simulink model "SR25"  (R2024a)
settings: Solver=FixedStepDiscrete  StartTime=0.0  StopTime=5  FixedStep=0.01  RelTol=1e-3  EnableMultiTasking=on
PreLoadFcn:
  | try, model_open; catch, disp('Error occurred while executing model pre-load callback: model_open.m'); disp('Please assure that the MATLAB working directory is set to the model directory before opening.'); end
InitFcn:
  | try, model_open; catch, end
undefined symbols (not defined in the file or in its folder): dt, GCM, raptor_get_safe_string, raptor_xcp_function
libraries: Raptor_lib x40, Utilities x13, TireTemperature x12, simulink x5, IO x5, APPS_BSPC x4, RotorTemperature x4, FlowRate x3, Cooling x2, BMS x2, Brakes x2, StateMachine x2
(part 1 of 3)
CloseFcn:
  | try, model_close; catch, end
settings Model: DataDictionary=SR25.sldd  Raptor_Target=GCM-1793-196-1503  Raptor_Calloc=NonVolatile (EEPROM)  RaptorUIDSize=4  RaptorBuildNum=100  Raptor_ecuaddr=11  Raptor_IsLiteMode=0  RaptorFaultManager=Standard  RaptorFaultManagerAddXYCounts=1  Creator=Ben  LastModifiedBy=msufs
settings SolverCC: AlgebraicLoopSolver=TrustRegion
settings DataIOCC: LimitDataPoints=on  SaveFormat=Array  SignalLoggingSaveFormat=ModelDataLogs  ReturnWorkspaceOutputs=off
settings OptimizationCC: DefaultParameterBehavior=Inlined  DefaultUnderspecifiedDataType=single  ReuseModelBlockBuffer=off  ExpressionDepthLimit=2147483647  InitFltsAndDblsToZero=on  LifeSpan=1  EfficientTunableParamExpr=on
settings DebuggingCC: SolverPrmCheckMsg=warning  InheritedTsInSrcMsg=none  FcnCallInpInsideContextMsg=warning  UnconnectedInputMsg=warning  UnconnectedOutputMsg=warning  UnconnectedLineMsg=warning  StateNameClashWarn=warning  SFUnexpectedBacktrackingDiag=warning  SFNoUnconditionalDefaultTransitionDiag=warning  SFExecutionAtInitializationDiag=none  ArithmeticOperatorsInVariantConditions=warning
settings HardwareCC: ProdBitPerPointer=32  ProdBitPerSizeT=32  ProdBitPerPtrDiffT=32  ProdLargestAtomicFloat=None  ProdWordSize=32  ProdHWDeviceType=Infineon->TriCore  TargetIntDivRoundTo=Zero  TargetEndianess=LittleEndian  TargetHWDeviceType=Infineon->TriCore  ProdEqTarget=off
settings ModelReferenceCC: EnableRefExpFcnMdlSchedulingChecks=on  PropagateSignalLabelsOutOfModel=off
settings SFSimCC: SimUseLocalCustomCode=off  MATLABDynamicMemAlloc=off  CustomCodeUndefinedFunction=UseInterfaceOnly
settings RTWCC: Description=Raptor (tm)  SystemTargetFile=raptor.tlc  MakeCommand=raptor_make_rtw  TemplateMakefile=raptor_GCM_1793_196_GCC.tmf  RTWUseLocalCustomCode=off  GPUComputeCapability=3.5
settings CodeAppCC: IgnoreCustomStorageClasses=off  MaxIdLength=100  CustomSymbolStrType=$N$R$M  StateflowObjectComments=on  InternalIdentifier=Classic
settings STFCustomTargetCC: TargetLangStandard=C89/C90 (ANSI)  CodeReplacementLibrary=GCM196-specific  GenerateSampleERTMain=on  CombineOutputUpdateFcns=on  ERTCustomFileBanners=on  SupportContinuousTime=off  SupportNonInlinedSFcns=off  RemoveResetFunc=on  MATLABClassNameForMDSCustomization=Simulink.SoftwareTarget.ERTCustomization  GRTInterface=off  UseToolchainInfoCompliant=off  SystemTargetFile=raptor.tlc
settings ERTTargetCC: CodeReplacementLibrary=GCM196-specific  MultiwordLength=2048  GenerateSampleERTMain=on  ParMdlRefBuildCompliant=off  CompOptLevelCompliant=off  ConcurrentExecutionCompliant=off  ModelStepFunctionPrototypeControlCompliant=off  CPPClassGenCompliant=off  UseToolchainInfoCompliant=off  ExtModeMexFile=noextcomm  InlinedParameterPlacement=NonHierarchical  ERTCustomFileTemplate=example_file_process.tlc  ConvertIfToSwitch=off  SuppressUnreachableDefaultCases=off
settings ConfigComp: CovMetricSettings=dw  CovSaveCumulativeToWorkspaceVar=on  CovSaveSingleToWorkspaceVar=on  CovExternalEMLEnable=off  CovSFcnEnable=off

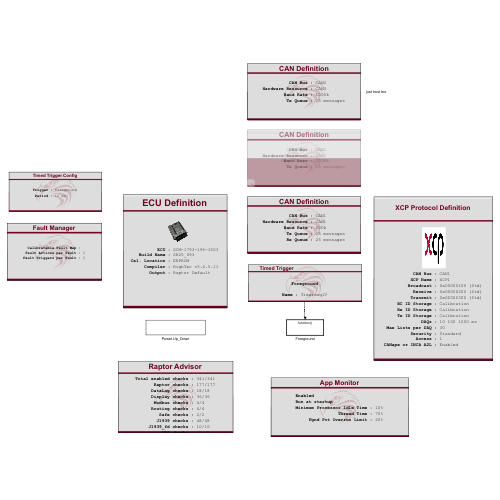
[thumbnail: Simulink's stored preview of the top-level diagram]
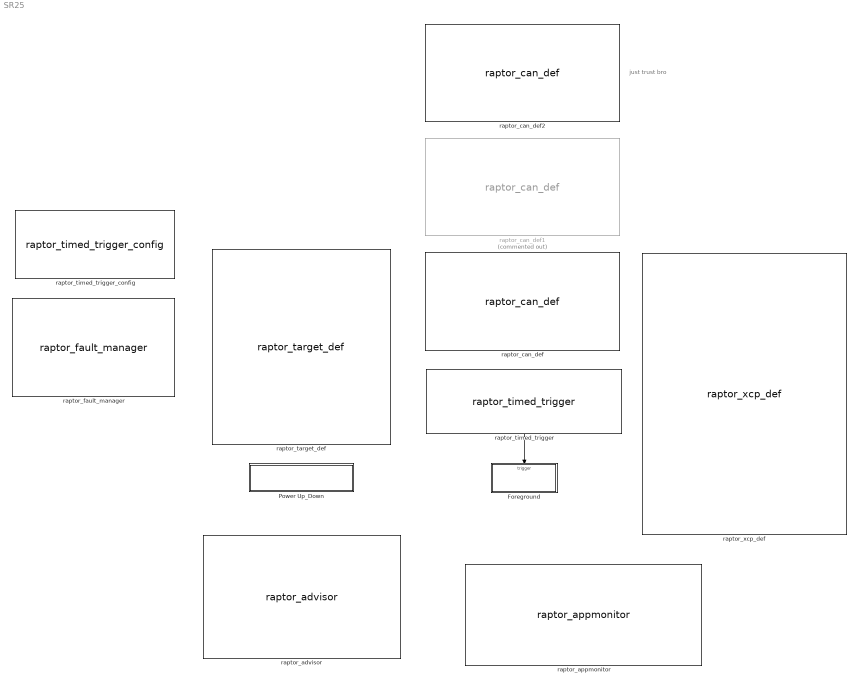
== system SR25 ==
  note: just trust bro
  Foreground : Subsystem  TreatAsAtomicUnit=on
      settings: RTWSystemCode=Nonreusable function
  Power Up_Down : Subsystem  mask{group='Diagnostics | Power Up_Down'}
  raptor_advisor : Raptor_lib/Configuration/raptor_advisor  pop_setEnable=Enable All  ckb_Raptor=on  ckb_AppMonitor=on  tbl_AppMonitor={ 'on', 'App Monitor'; 'on', 'App Monitor Measurement'; 'on', 'App Monitor Stop'; 'on', 'Reboot'; 'on', 'Task Monitor'; 'on', 'Task Monitor Measurement' }  ckb_CAN=on  tbl_CAN={ 'on', 'CAN Baud Rate'; 'on', 'CAN Bus Off Recovery'; 'on', 'CAN Definition'; 'on', 'CAN Hardware Mailbox Config'; 'on', 'CAN Mailbox Properties'; 'on', 'CAN Partial Networking'; 'on', 'CAN Queue Info'; 'on', 'CAN Rx Message'; 'on', 'CAN Rx Raw'; 'on', 'CAN State'; 'on', 'CAN Trigger'; 'on', 'CAN Tx Message'; 'on', 'CAN Tx Raw'; 'on', 'CAN/FD Definition'; 'on', 'CAN/FD Rx Message'; 'on', 'CAN/FD Rx Raw'; 'on', 'CAN/FD Tx Message'; 'on', 'CAN/FD Tx Raw'; 'on', 'Custom Baud Rate'; 'on', 'DBC Pack'; 'on', 'DBC Unpack' }  ckb_Checksum=on  tbl_Checksum={ 'on', 'Calculate Checksum'; 'on', 'Read Checksum' }  ckb_Config=on  tbl_Config={ 'on', 'Configuration Read'; 'on', 'ECU Definition'; 'on', 'Set Target Address'; 'on', 'System Variable Access Level'; 'on', 'XCP Custom Security Seed/Key'; 'on', 'XCP Custom Security Trigger'; 'on', 'XCP Protocol Definition'; 'on', 'XCP Query'; 'on', 'XCP Set Address' }  ckb_DataStore=on  tbl_DataStore={ 'on', 'Adjustment'; 'on', 'Data Read'; 'on', 'Data Store'; 'on', 'Data Write'; 'on', 'Fixed NV Manager'; 'on', 'Fixed NonVolatile Status'; 'on', 'Load NonVolatile Defaults'; 'on', 'Measurement'; 'on', 'Memory Read'; 'on', 'NonVolatile Settings'; 'on', 'NonVolatile Status'; 'on', 'Override'; 'on', 'Store NonVolatile' }  ckb_Engine=on  tbl_Engine={ 'on', 'Angle Time'; 'on', 'CamShaft Sensor Info'; 'on', 'Encoder Def'; 'on', 'Injector Output'; 'on', 'Knock Input'; 'on', 'Knock Results'; 'on', 'Spark Output'; 'on', 'Wideband O2 Input' }  ckb_Ethernet=on  tbl_Ethernet={ 'on', 'Ethernet Adapter Get MAC Address'; 'on', 'Ethernet Definition'; 'on', 'Ethernet Interface Definition'; 'on', 'Ethernet Interface Get VLAN'; 'on', 'Ethernet Interface Set VLAN'; 'on', 'Ethernet Socket - TCP Server'; 'on', 'Ethernet Socket - UDP Server'; 'on', 'Ethernet Socket State'; 'on', 'Ethernet TCP Accept'; 'on', 'Ethernet TCP Close'; 'on', 'Ethernet TCP Connect'; 'on', 'Ethernet TCP Listen'; 'on', 'Ethernet TCP Receive'; 'on', 'Ethernet TCP Send'; 'on', 'Ethernet TCP Shutdown'; 'on', 'Ethernet UDP Multicast Join'; 'on', 'Ethernet UDP Multicast Leave'; 'on', 'Ethernet UDP Receive'; 'on', 'Ethernet UDP Send' }  ckb_OBD_Faults=on  tbl_OBD_Faults={ 'on', 'Drive Cycle Complete'; 'on', 'Increment OBD Counter'; 'on', 'Increment OBD Ratio'; 'on', 'OBD Counter'; 'on', 'OBD Ratio'; 'on', 'Read OBD Counter'; 'on', 'Read OBD Ratio'; 'on', 'Reset OBD Counter'; 'on', 'Reset OBD Ratio' }  ckb_Faults=on  tbl_Faults={ 'on', 'Clear Fault'; 'on', 'Fault'; 'on', 'Fault Action'; 'on', 'Fault Action Iterator'; 'on', 'Fault Action Read'; 'on', 'Fault Config'; 'on', 'Fault Data'; 'on', 'Fault Data Read'; 'on', 'Fault Data Write'; 'on', 'Fault Handle'; 'on', 'Fault Iterator'; 'on', 'Fault Manager'; 'on', 'Fault Measurement'; 'on', 'Fault Reference'; 'on', 'Fault State Count'; 'on', 'Fault State Iterator'; 'on', 'Fault Status'; 'on', 'Fault Trigger'; 'on', 'Null Fault'; 'on', 'Set Fault State' }  ckb_IO=on  tbl_IO={ 'on', 'Analog Input'; 'on', 'Analog Input Reference'; 'on', 'Analog Output'; 'on', 'Device Diagnostics'; 'on', 'Digital Input'; 'on', 'Digital Output'; 'on', 'Frequency Input'; 'on', 'H-Bridge Output'; 'on', 'IMU Calibrate'; 'on', 'IMU Reset'; 'on', 'IMU Status'; 'on', 'Inertial Measurement'; 'on', 'Input Capture Defn'; 'on', 'Input Capture Get'; 'on', 'Input Capture Trigger'; 'on', 'Input Status'; 'on', 'Internal Measurement'; 'on', 'Output Status'; 'on', 'PWM Output'; 'on', 'Quadrature Input'; 'on', 'Set Hardware Option'; 'on', 'Set Input Option'; 'on', 'Temperature Measurement' }  ckb_LIN=on  tbl_LIN={ 'on', 'LIN Get Schedule'; 'on', 'LIN Master Definition'; 'on', 'LIN Rx Message'; 'on', 'LIN Set Schedule'; 'on', 'LIN Slave Definition'; 'on', 'LIN State'; 'on', 'LIN Trigger'; 'on', 'LIN Tx Message' }  ckb_SENT=on  tbl_SENT={ 'on', 'SENT Definition'; 'on', 'SENT Receive State' }  ckb_Serial=on  tbl_Serial={ 'on', 'Serial Definition'; 'on', 'Serial Rx'; 'on', 'Serial Trigger'; 'on', 'Serial Tx' }  ckb_Strings=on  tbl_Strings={ 'on', 'Arr 2 Str'; 'on', 'Printf'; 'on', 'Str 2 Arr'; 'on', 'String'; 'on', 'String Length'; 'on', 'String Reference'; 'on', 'scanf' }  ckb_Tables=on  tbl_Tables={ 'on', 'Axis'; 'on', 'Axis Reference'; 'on', 'Table Adapt'; 'on', 'Table Interpolate 1D'; 'on', 'Table Interpolate 1D Reference'; 'on', 'Table Interpolate 2D'; 'on', 'Table Interpolate 2D Reference' }  ckb_Time=on  tbl_Time={ 'on', 'Datetime Conversion In'; 'on', 'Datetime Conversion Out'; 'on', 'Real Time Clock Read'; 'on', 'Real Time Clock Set' }  ckb_Triggers=on  tbl_Triggers={ 'on', 'App Trigger'; 'on', 'Define Trigger'; 'on', 'Distributed Action Defn'; 'on', 'Distributed Action Execute'; 'on', 'Distributed Action Trigger'; 'on', 'Output Trigger Reference'; 'on', 'Shutdown'; 'on', 'Sleep'; 'on', 'Startup'; 'on', 'Time'; 'on', 'Timed Trigger'; 'on', 'Timed Trigger Config'; 'on', 'Trigger Execute'; 'on', 'Trigger Select'; 'on', 'dT' }  ckb_DataLog=on  tbl_DataLog={ 'on', 'Data Log Erase'; 'on', 'Data Log Read'; 'on', 'Data Log Write'; 'on', 'File Close'; 'on', 'File EOF'; 'on', 'File Exists'; 'on', 'File Get Free Space'; 'on', 'File Open'; 'on', 'File Position'; 'on', 'File Read'; 'on', 'File Remove'; 'on', 'File Rename'; 'on', 'File Seek'; 'on', 'File Size'; 'on', 'File Sync'; 'on', 'File Write'; 'on', 'USB Eject'; 'on', 'USB Status' }  ckb_Display=on  ckb_Drawing=on  tbl_Drawing={ 'on', 'Clear Rect'; 'on', 'Clear Screen'; 'on', 'Draw Arc'; 'on', 'Draw Button'; 'on', 'Draw Circle'; 'on', 'Draw Image'; 'on', 'Draw Line'; 'on', 'Draw Polygon'; 'on', 'Draw Rectangle'; 'on', 'Draw Text'; 'on', 'Element'; 'on', 'Fill Circle'; 'on', 'Fill Ellipse'; 'on', 'Fill Polygon'; 'on', 'Fill Rect'; 'on', 'Image Ref' }  ckb_Menu=on  tbl_Menu={ 'on', 'Menu Screen Definition'; 'on', 'Menu Sel Item'; 'on', 'Menu Text'; 'on', 'Menu Title' }  ckb_Prefab=on  tbl_Prefab={ 'on', 'Gauge: Create'; 'on', 'Gauge: Update' }  ckb_ScreenFuncs=on  tbl_ScreenFuncs={ 'on', 'Button Bar Properties'; 'on', 'Goto Screen'; 'on', 'Hide Buttonbar'; 'on', 'Recalibrate Screen'; 'on', 'Screen Definition'; 'on', 'Screen Reference'; 'on', 'Screen Select'; 'on', 'Setup Button'; 'on', 'Splash Screen' }  ckb_Touchscreen=on  tbl_Touchscreen={ 'on', 'Button Def'; 'on', 'Button Status'; 'on', 'Display Touchscreen'; 'on', 'Hot Area Actions'; 'on', 'Update Swipe Action' }  ckb_Modbus=on  tbl_Modbus={ 'on', 'Modbus Master'; 'on', 'Modbus Slave'; 'on', 'Modbus Slave Error'; 'on', 'Modbus Slave Response' }  ckb_Routing=on  tbl_Routing={ 'on', 'J1939 Message Router'; 'on', 'Message Hardware Filter'; 'on', 'Message Network'; 'on', 'Message Router' }  ckb_Safe=on  tbl_Safe={ 'on', 'Raptor Stack Check'; 'on', 'Raptor Time Check' }  ckb_J1939=on  ckb_DMA=on  tbl_DMA={ 'on', 'DM14/15/16 Definition: DM14 Rx'; 'on', 'DM14/15/16 Definition: DM15 Rx'; 'on', 'DM14/15/16 Definition: DM15 Tx'; 'on', 'DM14/15/16 Definition: DMA Manager'; 'on', 'DMA Address Space Definition'; 'on', 'DMA Address Space Return'; 'on', 'DMA Address Space Trigger'; 'on', 'DMA Key'; 'on', 'DMA Key Trigger' }  ckb_DM_Msgs=on  tbl_DM_Msgs={ 'on', 'DM19 Transmit'; 'on', 'DM20 Transmit'; 'on', 'DM21 Transmit'; 'on', 'DM22 Rx Trigger'; 'on', 'DM24 Transmit'; 'on', 'DM25 Transmit'; 'on', 'DM26 Transmit'; 'on', 'DM29 Transmit'; 'on', 'DM30 Transmit'; 'on', 'DM33 Transmit'; 'on', 'DM34 Transmit'; 'on', 'DM4 Transmit'; 'on', 'DM5 Transmit'; 'on', 'DM8 Transmit'; 'on', 'DTC Transmit' }  ckb_EFF=on  tbl_EFF={ 'on', 'Clear Expanded FF'; 'on', 'Expanded FF Status'; 'on', 'Write Expanded FF' }  ckb_PGN_Tx=on  tbl_PGN_Tx={ 'on', 'CBI Transmit'; 'on', 'CI Transmit'; 'on', 'EC1 Transmit'; 'on', 'ECUID Transmit'; 'on', 'GTFI Transmit'; 'on', 'LTFI Transmit'; 'on', 'RC Transmit'; 'on', 'SOFT Transmit'; 'on', 'TTI2 Transmit'; 'on', 'VI Transmit' }  ckb_SPN=on  tbl_SPN={ 'on', 'SPN Read'; 'on', 'SPN Write' }  ckb_J1939_TP=on  tbl_J1939_TP={ 'on', 'J1939 DTC Rx Handler'; 'on', 'J1939 Protocol'; 'on', 'J1939 Transport Protocol Receive'; 'on', 'PGN Enable'; 'on', 'PGN Request Slot'; 'on', 'PGN Rx Trigger'; 'on', 'PGN Trigger'; 'on', 'Source Addr'; 'on', 'Tx ACK/NACK' }  ckb_J1939_fd=on  ckb_J1939_fd_TP=on  tbl_J1939_fd_TP={'on','Get J1939 STD/FD Channel Addr.';'on','Rx Raw';'on','Transport Protocol';'on','Tx Raw'}  ckb_J1939_fd_GW=on  tbl_J1939_fd_GW={ 'on', 'Gateway'; 'on', 'Gateway Link'; 'on', 'Gateway Link Reset Stats'; 'on', 'Gateway Link Stats'; 'on', 'Gateway Network' }  ckb_UDS=on  ckb_ISO14229=on  tbl_ISO14229={ 'on', 'ISO14229 Custom Service 0x31'; 'on', 'ISO14229 Service 0x10 - Session Control'; 'on', 'ISO14229 Service 0x11 - ECU Reset'; 'on', 'ISO14229 Service 0x14 - Clear Diagnostic Information'; 'on', 'ISO14229 Service 0x19 - Extended Data Definition'; 'on', 'ISO14229 Service 0x19 - Read DTC Information'; 'on', 'ISO14229 Service 0x19 - Snapshot Record Clear'; 'on', 'ISO14229 Service 0x19 - Snapshot Record Clear All'; 'on', 'ISO14229 Service 0x19 - Snapshot Record Definition'; 'on', 'ISO14229 Service 0x19 - Snapshot Record Get'; 'on', 'ISO14229 Service 0x19 - Snapshot Record Set'; 'on', 'ISO14229 Service 0x22 - Read Data by Identifier'; 'on', 'ISO14229 Service 0x27 - Security Access'; 'on', 'ISO14229 Service 0x28 - Communication Control'; 'on', 'ISO14229 Service 0x2E - Write Data by Identifier'; 'on', 'ISO14229 Service 0x2F - Input Output by Identifier'; 'on', 'ISO14229 Service 0x2F - Input Output by Identifier Reset State'; 'on', 'ISO14229 Service 0x31 - Routine Control by Identifier'; 'on', 'ISO14229 Service 0x85 - DTC Control Setting' }  ckb_ISO15031=on  tbl_ISO15031={ 'on', 'ISO15031 Custom Service'; 'on', 'ISO15031 Service 0x01'; 'on', 'ISO15031 Service 0x03 - Emission-related diagnostic trouble codes'; 'on', 'ISO15031 Service 0x04 - Clear Diagnostic Information'; 'on', 'ISO15031 Service 0x07 - Emission-related pending diagnostic trouble codes'; 'on', 'ISO15031 Service 0x09 - Calibration Identification'; 'on', 'ISO15031 Service 0x09 - Calibration Verification Numbers'; 'on', 'ISO15031 Service 0x09 - ECU Name'; 'on', 'ISO15031 Service 0x09 - Request Vehicle Information'; 'on', 'ISO15031 Service 0x09 - Vehicle Identification Number'; 'on', 'ISO15031 Service 0x0A - Emission-related diagnostic trouble codes with permanent status' }  ckb_ISO15765=on  tbl_ISO15765={ 'on', 'ISO15765 Protocol Receive Queue Info'; 'on', 'ISO15765 Protocol Transmit Queue Info'; 'on', 'ISO15765 Protocol Transmit Raw' }  ckb_UDS_Basics=on  tbl_UDS_Basics={ 'on', 'UDS Client Functional Address Request'; 'on', 'UDS Client Functional Address Request Send'; 'on', 'UDS Protocol Client Request Raw'; 'on', 'UDS Protocol Receive Raw'; 'on', 'UDS Protocol Transmit Raw'; 'on', 'UDS Server Service Process Raw' }  ckb_UDS_Other=on  tbl_UDS_Other={ 'on', 'ISO13400 DoIP Entity'; 'on', 'UDS Protocol'; 'on', 'UDS Set Buffer Storage' }  ckb_J1939_Assure=on  tbl_J1939_Assure={ 'on', 'J1939-91C Network Config' }
      settings: SourceProductName=Raptor
  raptor_appmonitor : Raptor_lib/Application Monitoring/raptor_appmonitor  enabled=on  startupAction=Run  addStartupActionCal=off  minIdle=10  maxThread=70  calAccess=1  pctOverrunLimit=20  overrunAction=Stop Application  pauseOnReset=off  maxStackUsage=90  stackOverrunAction=Stop Application  addMaxStackCal=off  CANen=off
      settings: SourceProductName=Raptor
  raptor_can_def : Raptor_lib/CAN/raptor_can_def  canBus='CAN1'  resourceValues=CAN1|CAN2|CAN3|(None)  resource=CAN1  baudRateValues=125k|250k|500k|1000k  baudRate=500k  useCustomBR=0  customBR='CustomBaudRate'  enable_baud_rate_config='RAPTOR MASK DEFAULT'  sim_func_name='RAPTOR MASK DEFAULT'  createButton=[]  updateButton=[]  txQueueSize=25  rxQueueSize=25
      settings: SourceProductName=Raptor
  raptor_can_def1 : Raptor_lib/CAN/raptor_can_def  Commented=on  canBus='CAN2'  resourceValues=CAN1|CAN2|CAN3|(None)  resource=CAN2  baudRateValues=125k|250k|500k|1000k  baudRate=1000k  useCustomBR=0  customBR='CustomBaudRate'  enable_baud_rate_config='RAPTOR MASK DEFAULT'  sim_func_name='RAPTOR MASK DEFAULT'  createButton=[]  updateButton=[]  txQueueSize=25  rxQueueSize=22
      settings: SourceProductName=Raptor
  raptor_can_def2 : Raptor_lib/CAN/raptor_can_def  canBus='CAN2'  resourceValues=CAN1|CAN2|CAN3|(None)  resource=CAN3  baudRateValues=125k|250k|500k|1000k  baudRate=1000k  useCustomBR=0  customBR='CustomBaudRate'  enable_baud_rate_config='RAPTOR MASK DEFAULT'  sim_func_name='RAPTOR MASK DEFAULT'  createButton=[]  updateButton=[]  txQueueSize=25  rxQueueSize=22
      settings: SourceProductName=Raptor
  raptor_fault_manager : Raptor_lib/Faults/raptor_fault_manager  button=0  managerTypeValues=Standard|OBD  managerType=Standard  cyclesToHeal=3  cyclesToClear=40  addXYCounts=1  calFaultMap=1  minFaultActions=2  minFaultTriggers=2  calAccessValues=4|3|2|1  calAccess=1  calFunction='System | FaultManager'  initMap=struct('managerType', 'Standard','actionMap', {{struct('fault', 'APPSFault','action', 'TorqueCmdOverride','state', [ 4;]),struct('fault', 'BSPCTriggerFault','action', 'TorqueCmdOverride','state', [ 4;]),struct('fault', 'BSPCTriggerFault','action', 'TorqueCmdOverride','state', [ 8;]),struct('fault', 'CTRL_SegmentOverTempFault','action', 'VehicleFault','state', [ 4;]),struct('fault', 'CTRL_SegmentOverVoltFault','action', 'VehicleFault','state', [ 4;]),struct('fault', 'CTRL_SegmentUnderTempFault','action', 'VehicleFault','state', [ 4;]),struct('fault', 'CTRL_SegmentUnderVoltFault','action', 'VehicleFault','state', [ 4;]),struct('fault', 'IN_BrakePressureFFault','action', 'TorqueCmdOverride','state', [ 4;]),struct('fault', 'IN_BrakePressureFFault','action', 'TorqueCmdOverride','state', [ 8;]),struct('fault', 'IN_BrakePressureRFault','action', 'TorqueCmdOverride','state', [ 4;]),struct('fault', 'IN_BrakePressureRFault','action', 'TorqueCmdOverride','state', [ 8;]),struct('fault', 'IN_CAN1_160_Fault','action', 'TorqueCmdOverride','state', [ 4;]),struct('fault', 'IN_CAN1_160_Fault','action', 'TorqueCmdOverride','state', [ 8;]),struct('fault', 'IN_CAN1_162_Fault','action', 'TorqueCmdOverride','state', [ 4;]),struct('fault', 'IN_CAN1_162_Fault','action', 'TorqueCmdOverride','state', [ 8;]),struct('fault', 'IN_CAN1_167_Fault','action', 'TorqueCmdOverride','state', [ 4;]),struct('fault', 'IN_CAN1_167_Fault','action', 'TorqueCmdOverride','state', [ 8;]),struct('fault', 'IN_ThrottlePosition1Fault','action', 'TorqueCmdOverride','state', [ 4;]),struct('fault', 'IN_ThrottlePosition1Fault','action', 'TorqueCmdOverride','state', [ 8;]),struct('fault', 'IN_ThrottlePosition2Fault','action', 'TorqueCmdOverride','state', [ 4;]),struct('fault', 'IN_ThrottlePosition2Fault','action', 'TorqueCmdOverride','state', [ 8;])}},'triggerMap', {{}})  exportFilePath='C:\'  exportFileName='FaultMapExport_01.csv'
      settings: SourceProductName=Raptor
  raptor_target_def : Raptor_lib/Configuration/raptor_target_def  targetValues=CCM-58NN-112-2403|DISP-VC128-1901|DISP-VC320L-1402|DISP-VC320-1204|DISP-VC800-1402|DISP-VC500-1904|DISP-VC700-2003|DISP-VC300R-2004|GCM-5634M-070-1559|GCM-5634M-070-1562|EOL-58NN-176-2204|ECM-1793-196-1503|GCM-1793-196-1503|GCM-5605B-048-1906|GCM-5605B-048-2104|RCM-5743R-080-2203|RCM-5743R-080-2304|UAS-5743R-047-2102|UAS-5743R-047-2107|RCM-58NN-112-2103|RCM-58NN-112-2202|RCM-58NN-112-2208|RCM-58NN-112-2210|GCM-TC337-056-2402|GCM-TC367-111-2301|HCM-5604-036-1303|HCM-5604-036-1702  target=GCM-1793-196-1503  simpack=0  simulator=0  heap=4*1024  stack=2*1024  fgndStack=3*1024  bgndStack=2*1024  idleStack=1024  intStack=1536  sdStack=1024  appStack=1024  ecuaddr=11  uds_server_addr_ext=0  uds_server_addr=hex2dec('600')  uds_client_addr=hex2dec('650')  callocValues=Constant (FLASH)|NonVolatile (EEPROM)  calloc=NonVolatile (EEPROM)  compilerValues=HighTec v3.4.5.11  compiler=HighTec v3.4.5.11  setFileName=0  exeName=[raptor_get_safe_string(bdroot) '_']  addBuildNum=1  minVerChars=3  extraOutput=1  buildLocationValues=Raptor Default|Model Directory|User Defined  buildLocation=Raptor Default  exeLocation=''  exeFileButton=0  a2lLocation=''  a2lFileButton=0  rpgLocation=''  rpgFileButton=0
      settings: SourceProductName=Raptor
  raptor_timed_trigger : Raptor_lib/Triggers/raptor_timed_trigger  triggerValues=Foreground|Foregroundx2|Foregroundx5|Foregroundx10|Foregroundx20|Background|Backgroundx2|Backgroundx5|Backgroundx10|Backgroundx20|Second|Minute|Task_1ms  trigger=Foreground  inherited=0  alwaysEnabled=1  triggerPriority=0  triggerName=ooqlV
      settings: SourceProductName=Raptor
  raptor_timed_trigger_config : Raptor_lib/Triggers/raptor_timed_trigger_config  triggerValues=Foreground|Background|Second|Minute  trigger=Foreground  period=10
      settings: SourceProductName=Raptor
  raptor_xcp_def : Raptor_lib/Configuration/raptor_xcp_def  XCPname='XCP1'  canBus='CAN1'  bcID=hex2dec('100')  bcID_TypeValues=Standard|Extended  bcID_Type=Standard  rxID=hex2dec('200')  rxID_TypeValues=Standard|Extended  rxID_Type=Standard  txID=hex2dec('300')  txID_TypeValues=Standard|Extended  txID_Type=Standard  daqRates=[10 100 1000]  numODTs=30  genCANAPE=1  genVISION=0  securityValues=Standard|None|Custom User Defined  security=Standard  dllName=raptor_XCPSecurity.dll  accessValues=4|3|2|1  access=1  bcStorageValues=Constant (FLASH)|NonVolatile (EEPROM)|FixedNonVolatile (EEPROM)|Volatile (RAM)|Calibration  bcStorage=Calibration  txStorageValues=Constant (FLASH)|NonVolatile (EEPROM)|FixedNonVolatile (EEPROM)|Volatile (RAM)|Calibration  txStorage=Calibration  rxStorageValues=Constant (FLASH)|NonVolatile (EEPROM)|FixedNonVolatile (EEPROM)|Volatile (RAM)|Calibration  rxStorage=Calibration
      settings: SourceProductName=Raptor
  wires:
  raptor_timed_trigger/1 -> Foreground/Trigger

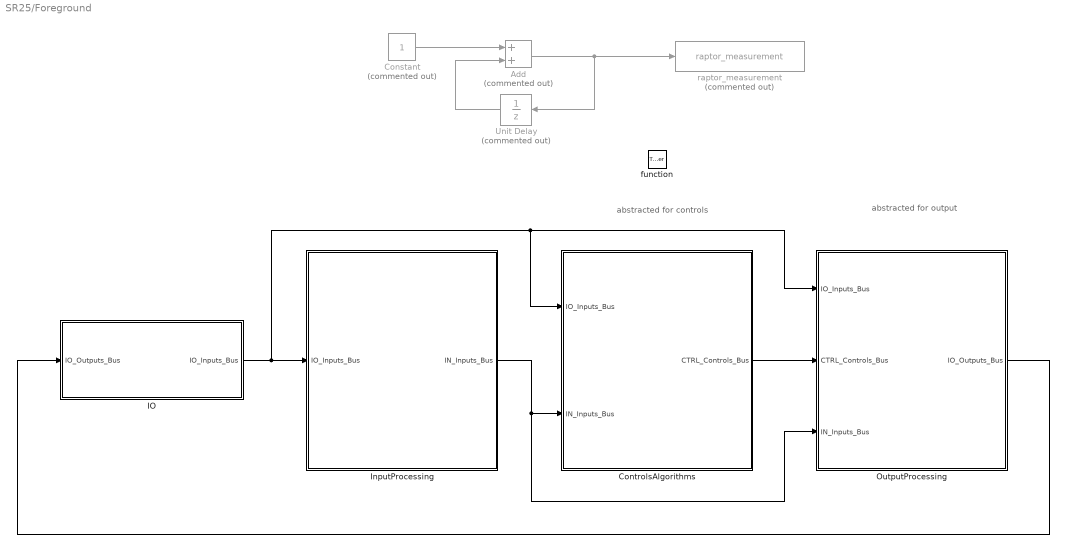
== system SR25/Foreground ==
  note: abstracted for output
  note: abstracted for controls
  function : TriggerPort  TriggerType=function-call  VariantControl=Variant
  Add : Sum  Commented=on
  Constant : Constant  Commented=on
  ControlsAlgorithms : Subsystem
  IO : Subsystem
  InputProcessing : Subsystem
  OutputProcessing : Subsystem
  Unit Delay : UnitDelay  Commented=on  SampleTime=-1  HasFrameUpgradeWarning=on
  raptor_measurement : Raptor_lib/Data Storage/raptor_measurement  Commented=on  paramName='Counter'  nameSource=Parameter  calDispType=Number  calEnum={'False', 'True'}  calGain=1.0  calOffset=0.0  calMax=inf  calMin=-inf  calFormat='-1'  calUnit=''  calHelp=''  calAccess=4  calFunction=raptor_xcp_function(gcb)  calVisible=on
      settings: SourceProductName=Raptor
  wires:
  Constant/1 -> Add/1
  Add/1 -> raptor_measurement/1, Unit Delay/1
  Unit Delay/1 -> Add/2
  InputProcessing/1(IN_Inputs_Bus) -> OutputProcessing/3(IN_Inputs_Bus), ControlsAlgorithms/2(IN_Inputs_Bus)
  IO/1(IO_Inputs_Bus) -> OutputProcessing/1(IO_Inputs_Bus), ControlsAlgorithms/1(IO_Inputs_Bus), InputProcessing/1(IO_Inputs_Bus)
  OutputProcessing/1(IO_Outputs_Bus) -> IO/1(IO_Outputs_Bus)
  ControlsAlgorithms/1(CTRL_Controls_Bus) -> OutputProcessing/2(CTRL_Controls_Bus)

== system SR25/Power Up_Down ==
  Background : Subsystem
  raptor_timed_trigger : Raptor_lib/Triggers/raptor_timed_trigger  triggerValues=Foreground|Foregroundx2|Foregroundx5|Foregroundx10|Foregroundx20|Background|Backgroundx2|Backgroundx5|Backgroundx10|Backgroundx20|Second|Minute|Task_1ms  trigger=Background  inherited=0  alwaysEnabled=1  triggerPriority=50  triggerName=BGND_G6Wyo
      settings: SourceProductName=Raptor
  wires:
  raptor_timed_trigger/1 -> Background/Trigger

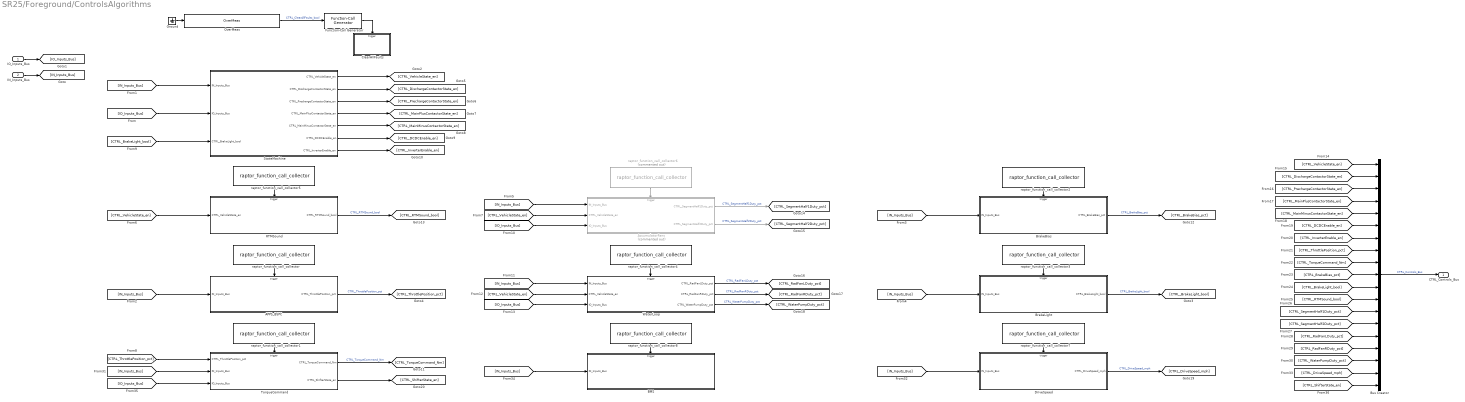
== system SR25/Foreground/ControlsAlgorithms ==
  IO_Inputs_Bus : Inport
  IN_Inputs_Bus : Inport  Port=2
  APPS_BSPC : Subsystem  TreatAsAtomicUnit=on
  AccumulatorFans : Subsystem  Commented=on  TreatAsAtomicUnit=on
  BMS : Subsystem  TreatAsAtomicUnit=on
  BrakeBias : Subsystem  TreatAsAtomicUnit=on
  BrakeLight : Subsystem  TreatAsAtomicUnit=on
  Bus Creator : BusCreator  Inputs=19
  ClearAllFaults : Subsystem  TreatAsAtomicUnit=on
  DriveSpeed : Subsystem  TreatAsAtomicUnit=on
  Function-Call Generator : simulink/Ports & Subsystems/Function-Call Generator  sample_time=1  numberOfIterations=1  DisallowWideOutput=off  ShowEnablePort=on
  Ground : Ground
  OverMeas : Utilities/OverMeas  sigName='CTRL_ClearAllFaults_bool'  minimum=0  maximum=1
  RTMSound : Subsystem  TreatAsAtomicUnit=on
  StateMachine : Subsystem
  TorqueCommand : Subsystem  TreatAsAtomicUnit=on
  WaterLoop : Subsystem  TreatAsAtomicUnit=on
  raptor_function_call_collector : Raptor_lib/Triggers/raptor_function_call_collector  count=1
      settings: SourceProductName=Raptor
  raptor_function_call_collector1 : Raptor_lib/Triggers/raptor_function_call_collector  count=1
      settings: SourceProductName=Raptor
  raptor_function_call_collector2 : Raptor_lib/Triggers/raptor_function_call_collector  count=100
      settings: SourceProductName=Raptor
  raptor_function_call_collector3 : Raptor_lib/Triggers/raptor_function_call_collector  count=10
      settings: SourceProductName=Raptor
  raptor_function_call_collector4 : Raptor_lib/Triggers/raptor_function_call_collector  count=100
      settings: SourceProductName=Raptor
  raptor_function_call_collector5 : Raptor_lib/Triggers/raptor_function_call_collector  count=10
      settings: SourceProductName=Raptor
  raptor_function_call_collector6 : Raptor_lib/Triggers/raptor_function_call_collector  Commented=on  count=100
      settings: SourceProductName=Raptor
  raptor_function_call_collector7 : Raptor_lib/Triggers/raptor_function_call_collector  count=10
      settings: SourceProductName=Raptor
  raptor_function_call_collector8 : Raptor_lib/Triggers/raptor_function_call_collector  count=100
      settings: SourceProductName=Raptor
  CTRL_Controls_Bus : Outport
  wires:
  [IN_Inputs_Bus] -> APPS_BSPC/1(IN_Inputs_Bus)
  raptor_function_call_collector/1 -> APPS_BSPC/Trigger
  APPS_BSPC/1(CTRL_ThrottlePosition_pct) -> [CTRL_ThrottlePosition_pct]  "CTRL_ThrottlePosition_pct"
  raptor_function_call_collector1/1 -> TorqueCommand/Trigger
  Bus Creator/1 -> CTRL_Controls_Bus/1  "CTRL_Controls_Bus"
  TorqueCommand/1(CTRL_TorqueCommand_Nm) -> [CTRL_TorqueCommand_Nm]  "CTRL_TorqueCommand_Nm"
  OverMeas/1 -> Function-Call Generator/1  "CTRL_ClearAllFaults_bool"
  Function-Call Generator/1 -> ClearAllFaults/Trigger
  Ground/1 -> OverMeas/1
  raptor_function_call_collector2/1 -> BrakeBias/Trigger
  BrakeBias/1(CTRL_BrakeBias_pct) -> [CTRL_BrakeBias_pct]  "CTRL_BrakeBias_pct"
  BrakeLight/1(CTRL_BrakeLight_bool) -> [CTRL_BrakeLight_bool]  "CTRL_BrakeLight_bool"
  raptor_function_call_collector3/1 -> BrakeLight/Trigger
  [IO_Inputs_Bus] -> StateMachine/2(IO_Inputs_Bus)
  StateMachine/1(CTRL_VehicleState_en) -> [CTRL_VehicleState_en]
  StateMachine/5(CTRL_MainMinusContactorState_en) -> [CTRL_MainMinusContactorState_en]
  StateMachine/4(CTRL_MainPlusContactorState_en) -> [CTRL_MainPlusContactorState_en]
  StateMachine/3(CTRL_PrechargeContactorState_en) -> [CTRL_PrechargeContactorState_en]
  StateMachine/2(CTRL_DischargeContactorState_en) -> [CTRL_DischargeContactorState_en]
  StateMachine/6(CTRL_DCDCEnable_en) -> [CTRL_DCDCEnable_en]
  StateMachine/7(CTRL_InverterEnable_en) -> [CTRL_InverterEnable_en]
  raptor_function_call_collector5/1 -> RTMSound/Trigger
  RTMSound/1(CTRL_RTMSound_bool) -> [CTRL_RTMSound_bool]  "CTRL_RTMSound_bool"
  raptor_function_call_collector6/1 -> AccumulatorFans/Trigger
  IO_Inputs_Bus/1 -> [IO_Inputs_Bus]
  IN_Inputs_Bus/1 -> [IN_Inputs_Bus]
  [IN_Inputs_Bus] -> StateMachine/1(IN_Inputs_Bus)
  [IN_Inputs_Bus] -> BrakeBias/1(IN_Inputs_Bus)
  [IN_Inputs_Bus] -> BrakeLight/1(IN_Inputs_Bus)
  [IN_Inputs_Bus] -> AccumulatorFans/1(IN_Inputs_Bus)
  [CTRL_VehicleState_en] -> RTMSound/1(CTRL_VehicleState_en)
  [CTRL_ThrottlePosition_pct] -> TorqueCommand/1(CTRL_ThrottlePosition_pct)
  [CTRL_BrakeLight_bool] -> StateMachine/3(CTRL_BrakeLight_bool)
  [CTRL_VehicleState_en] -> AccumulatorFans/2(CTRL_VehicleState_en)
  [IO_Inputs_Bus] -> AccumulatorFans/3(IO_Inputs_Bus)
  AccumulatorFans/1(CTRL_SegmentHalf1Duty_pct) -> [CTRL_SegmentHalf1Duty_pct]  "CTRL_SegmentHalf1Duty_pct"
  AccumulatorFans/2(CTRL_SegmentHalf2Duty_pct) -> [CTRL_SegmentHalf2Duty_pct]  "CTRL_SegmentHalf2Duty_pct"
  raptor_function_call_collector4/1 -> WaterLoop/Trigger
  [IN_Inputs_Bus] -> WaterLoop/1(IN_Inputs_Bus)
  [CTRL_VehicleState_en] -> WaterLoop/2(CTRL_VehicleState_en)
  [IO_Inputs_Bus] -> WaterLoop/3(IO_Inputs_Bus)
  WaterLoop/1(CTRL_RadFanLDuty_pct) -> [CTRL_RadFanLDuty_pct]  "CTRL_RadFanLDuty_pct"
  WaterLoop/2(CTRL_RadFanRDuty_pct) -> [CTRL_RadFanRDuty_pct]  "CTRL_RadFanRDuty_pct"
  WaterLoop/3(CTRL_WaterPumpDuty_pct) -> [CTRL_WaterPumpDuty_pct]  "CTRL_WaterPumpDuty_pct"
  [CTRL_VehicleState_en] -> Bus Creator/1
  [CTRL_DischargeContactorState_en] -> Bus Creator/2
  [CTRL_PrechargeContactorState_en] -> Bus Creator/3
  [CTRL_MainPlusContactorState_en] -> Bus Creator/4
  [CTRL_MainMinusContactorState_en] -> Bus Creator/5
  [CTRL_DCDCEnable_en] -> Bus Creator/6
  [CTRL_InverterEnable_en] -> Bus Creator/7
  [CTRL_ThrottlePosition_pct] -> Bus Creator/8
  [CTRL_TorqueCommand_Nm] -> Bus Creator/9
  [CTRL_BrakeBias_pct] -> Bus Creator/10
  [CTRL_BrakeLight_bool] -> Bus Creator/11
  [CTRL_RTMSound_bool] -> Bus Creator/12
  [CTRL_SegmentHalf1Duty_pct] -> Bus Creator/13
  [CTRL_SegmentHalf2Duty_pct] -> Bus Creator/14
  [CTRL_RadFanLDuty_pct] -> Bus Creator/15
  [CTRL_RadFanRDuty_pct] -> Bus Creator/16
  [CTRL_WaterPumpDuty_pct] -> Bus Creator/17
  [IN_Inputs_Bus] -> TorqueCommand/2(IN_Inputs_Bus)
  raptor_function_call_collector7/1 -> DriveSpeed/Trigger
  [IN_Inputs_Bus] -> DriveSpeed/1(IN_Inputs_Bus)
  DriveSpeed/1(CTRL_DriveSpeed_mph) -> [CTRL_DriveSpeed_mph]  "CTRL_DriveSpeed_mph"
  [CTRL_DriveSpeed_mph] -> Bus Creator/18
  raptor_function_call_collector8/1 -> BMS/Trigger
  [IN_Inputs_Bus] -> BMS/1(IN_Inputs_Bus)
  [IO_Inputs_Bus] -> TorqueCommand/3(IO_Inputs_Bus)
  TorqueCommand/2(CTRL_ShifterState_en) -> [CTRL_ShifterState_en]
  [CTRL_ShifterState_en] -> Bus Creator/19

== system SR25/Foreground/IO ==
  IO_Outputs_Bus : Inport
  Inputs : Subsystem
  Outputs : Subsystem
  IO_Inputs_Bus : Outport
  wires:
  Inputs/1(IO_Inputs_Bus) -> IO_Inputs_Bus/1
  IO_Outputs_Bus/1 -> Outputs/1(IO_Outputs_Bus)
